simulink model "dymanics_modelling_dc"  (R2022b)
settings: Solver=VariableStepAuto  StartTime=0.0  StopTime=10.0  RelTol=1e-3
settings Model: Creator=sokse  LastModifiedBy=sokse

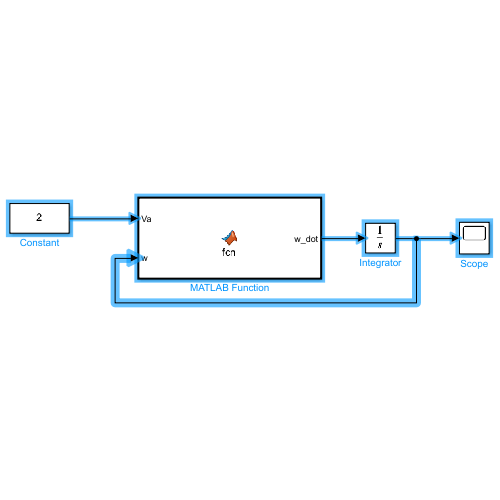
[thumbnail: Simulink's stored preview of the top-level diagram]
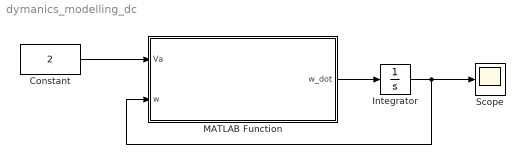
== system dymanics_modelling_dc ==
  Constant : Constant  Value=2
  Integrator : Integrator
  MATLAB Function : MATLAB Function  TreatAsAtomicUnit=on
  Scope : Scope
  wires:
  Constant/1 -> MATLAB Function/1(Va)
  MATLAB Function/1(w_dot) -> Integrator/1
  Integrator/1 -> MATLAB Function/2(w), Scope/1

== matlab function dymanics_modelling_dc/MATLAB Function ==
  data: Va input; w_dot output; w input
function w_dot = fcn(Va,w)

a = 10; 
b = 25; 
w_dot = -a*w+b*Va;
